simulink model "finger"  (R2020b)
settings: Solver=VariableStepAuto  StartTime=0.0  StopTime=4  FixedStep=0.0005  RelTol=1e-3  AbsTol=1e-3  EnableMultiTasking=on
values from neighbouring files (symbols this model uses):
  radius_finger = 0.031    [simulationv1.m]
  revolute_x = 0    [simulationv1.m]
  revolute_y = 0    [simulationv1.m]
  robot_height = 0.2    [simulationv1.m]
  robot_width = 0.6    [simulationv1.m]
  size_strut = 45 * 10^-3    (= 0.045)    [simulationv1.m]
  t_sample = 0.001    [simulationv1.m]
undefined symbols (not defined in the file or in its folder): climit, F_push, g_0, quarter_circle, sigbuilder_block, X, Y, Z
libraries: sm_lib x24, nesl_utility x11, pid_lib x3, dspstat3 x2, dspsigops x1, simulink x1
(part 2 of 2)

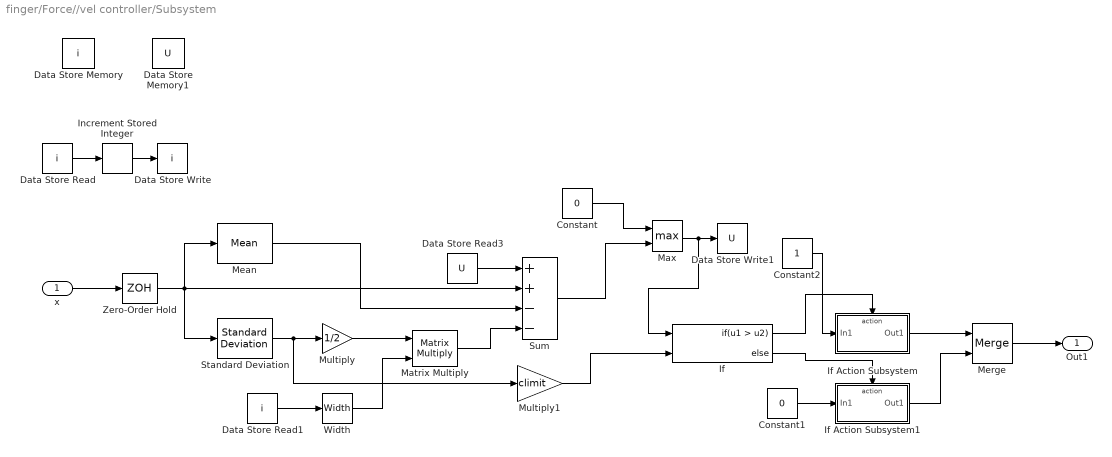
== system finger/Force//vel controller/Subsystem ==
  x : Inport
  Constant : Constant  Value=0
  Constant1 : Constant  Value=0
  Constant2 : Constant
  Data Store Memory : DataStoreMemory  DataStoreName=i  ReadBeforeWriteMsg=warning  WriteAfterWriteMsg=warning  WriteAfterReadMsg=warning  ShowAdditionalParam=off
  Data Store Memory1 : DataStoreMemory  DataStoreName=U  ReadBeforeWriteMsg=warning  WriteAfterWriteMsg=warning  WriteAfterReadMsg=warning  ShowAdditionalParam=off
  Data Store Read : DataStoreRead  DataStoreName=i
  Data Store Read1 : DataStoreRead  DataStoreName=i
  Data Store Read3 : DataStoreRead  DataStoreName=U
  Data Store Write : DataStoreWrite  DataStoreName=i
  Data Store Write1 : DataStoreWrite  DataStoreName=U
  If : If  NumInputs=2  IfExpression=u1 > u2
  If Action Subsystem : Subsystem  TreatAsAtomicUnit=on
  If Action Subsystem1 : Subsystem  TreatAsAtomicUnit=on
  Increment Stored Integer : simulink/Additional Math & Discrete/Additional Math: Increment - Decrement/Increment Stored Integer
  Matrix Multiply : Product  Multiplication=Matrix(*)
  Max : MinMax  Function=max  Inputs=2
  Mean : dspstat3/Mean  run=on  InputProcessing=Columns as channels (frame based)  reset_popup=None  directionMode=Each column  dimension=1  roiEnable=off  roiType=Rectangles  roiPortion=Entire ROI  roiOutput=Individual statistics for each ROI  roiFlag=off  roundingMode=Floor  overflowMode=off  outputDataTypeStr=Inherit: Same as accumulator  outputMin=[]  outputMax=[]  outputLastDataTypeStr=Inherit: Same as accumulator
  Merge : Merge
  Multiply : Gain  Gain=1/2
  Multiply1 : Gain  Gain=climit
  Standard Deviation : dspstat3/Standard Deviation  run=on  directionMode=Each column  dimension=1  InputProcessing=Columns as channels (frame based)  reset_popup=None  roiEnable=off  roiType=Rectangles  roiPortion=Entire ROI  roiOutput=Individual statistics for each ROI  roiFlag=off
      settings: SourceProductBaseCode=DS
  Sum : Sum  Inputs=++--
  Width : Width
  Zero-Order Hold : ZeroOrderHold  SampleTime=-1
  Out1 : Outport
  wires:
  Constant/1 -> Max/1
  Data Store Read3/1 -> Sum/1
  Mean/1 -> Sum/3
  Sum/1 -> Max/2
  Standard Deviation/1 -> Multiply1/1, Multiply/1
  Max/1 -> If/1, Data Store Write1/1
  Multiply/1 -> Matrix Multiply/1
  Matrix Multiply/1 -> Sum/4
  Width/1 -> Matrix Multiply/2
  Data Store Read/1 -> Increment Stored Integer/1
  Increment Stored Integer/1 -> Data Store Write/1
  Data Store Read1/1 -> Width/1
  Zero-Order Hold/1 -> Sum/2, Standard Deviation/1, Mean/1
  Multiply1/1 -> If/2
  If/1 -> If Action Subsystem/Action
  If Action Subsystem/1(Out1) -> Merge/1
  If Action Subsystem1/1(Out1) -> Merge/2
  If/2 -> If Action Subsystem1/Action
  Constant1/1 -> If Action Subsystem1/1(In1)
  Constant2/1 -> If Action Subsystem/1(In1)
  x/1 -> Zero-Order Hold/1
  Merge/1 -> Out1/1

== system finger/Force//vel controller/Subsystem/If Action Subsystem ==
  In1 : Inport
  Action Port : ActionPort  ActionPortLabel=if(u1 > u2)
  Out1 : Outport
  wires:
  In1/1 -> Out1/1

== system finger/Force//vel controller/Subsystem/If Action Subsystem1 ==
  In1 : Inport
  Action Port : ActionPort  ActionPortLabel=else
  Out1 : Outport
  wires:
  In1/1 -> Out1/1
